simulink model "SFverinsC"  (R2020a)
settings: Solver=VariableStepAuto  StartTime=0.0  StopTime=inf  RelTol=1e-5
libraries: simulink x5
settings Model: Creator=maxen  LastModifiedBy=maxen

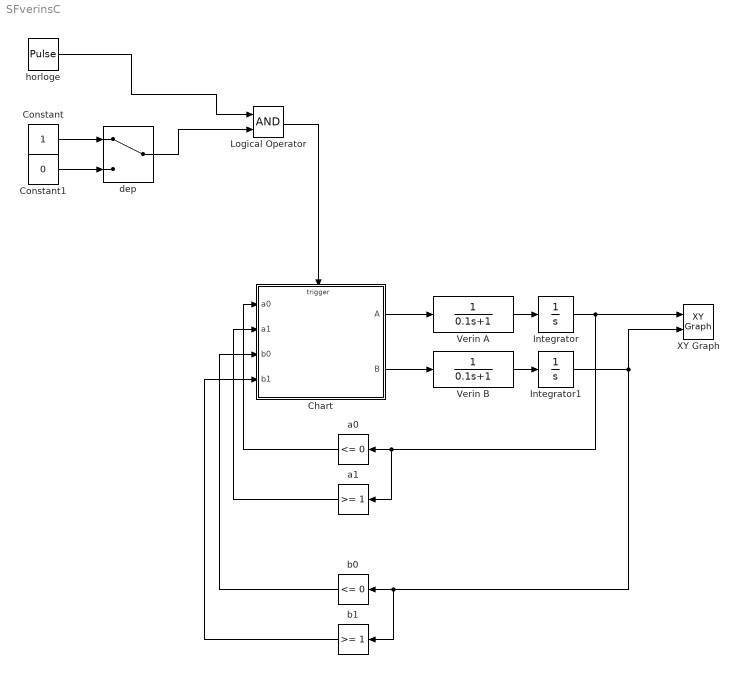
== system SFverinsC ==
  Chart : Stateflow chart  TreatAsAtomicUnit=on
  Constant : Constant
  Constant1 : Constant  Value=0
  Integrator : Integrator  InitialCondition=0.5
  Integrator1 : Integrator  InitialCondition=0.5
  Logical Operator : Logic  AllPortsSameDT=off  OutDataTypeStr=boolean
  Verin A : TransferFcn  Denominator=[0.1 1]
  Verin B : TransferFcn  Denominator=[0.1 1]
  XY Graph : simulink/Sinks/XY Graph  xmin=-2  xmax=2  ymin=-2  ymax=2  st=-1
  a0 : simulink/Logic and Bit Operations/Compare To Zero  relop=<=  OutDataTypeStr=boolean
  a1 : simulink/Logic and Bit Operations/Compare To Constant  relop=>=  const=1  OutDataTypeStr=boolean
  b0 : simulink/Logic and Bit Operations/Compare To Zero  relop=<=  OutDataTypeStr=boolean
  b1 : simulink/Logic and Bit Operations/Compare To Constant  relop=>=  const=1  OutDataTypeStr=boolean
  dep : ManualSwitch
  horloge : DiscretePulseGenerator  PulseType=Time based  Period=0.01  PulseWidth=5
  wires:
  Constant/1 -> dep/1
  Constant1/1 -> dep/2
  Chart/1(A) -> Verin A/1
  Chart/2(B) -> Verin B/1
  Verin A/1 -> Integrator/1
  Verin B/1 -> Integrator1/1
  Integrator/1 -> a1/1, a0/1, XY Graph/1
  Integrator1/1 -> XY Graph/2, b1/1, b0/1
  a0/1 -> Chart/1(a0)
  a1/1 -> Chart/2(a1)
  b0/1 -> Chart/3(b0)
  b1/1 -> Chart/4(b1)
  horloge/1 -> Logical Operator/1
  dep/1 -> Logical Operator/2
  Logical Operator/1 -> Chart/Trigger

== stateflow chart SFverinsC/Chart ==
  state Less_AB
    state B [parallel]
      settings: executionOrder=1
      state Less_B
        en:B=-1;
      state Less_B1
        en:B=0;
      (default) -> Less_B
      Less_B -> Less_B1 : [b0]
    state A [parallel]
      settings: executionOrder=2
      state Less_A
        en:A=-1;
      state Less_A1
        en:A=0;
      (default) -> Less_A
      Less_A -> Less_A1 : [a0]
  state Initial_State
  state Full_A
    en:A=1;
    en:B=0;
  state Full_B
    en:A=0;
    en:B=1;
  Less_AB -> Initial_State
  (default) -> Initial_State
  Initial_State -> Less_AB [order 2] : [~a0 || ~b0]
  Initial_State -> Full_A [order 1] : [dep && a0 && b0]
  Full_B -> Less_AB : [b1]
  Full_A -> Full_B : [a1]
  data: a0 input; a1 input; b0 input; b1 input; A output; B output
  events: dep input EITHER_EDGE_EVENT
